simulink model "VRcukie"  (R2013a)
settings: Solver=ode45  StartTime=0.0  StopTime=10.0  RelTol=1e-3
libraries: aerolibanimutils x1, vrlib x1
settings Model: Creator=Grompone  LastModifiedBy=Grompone

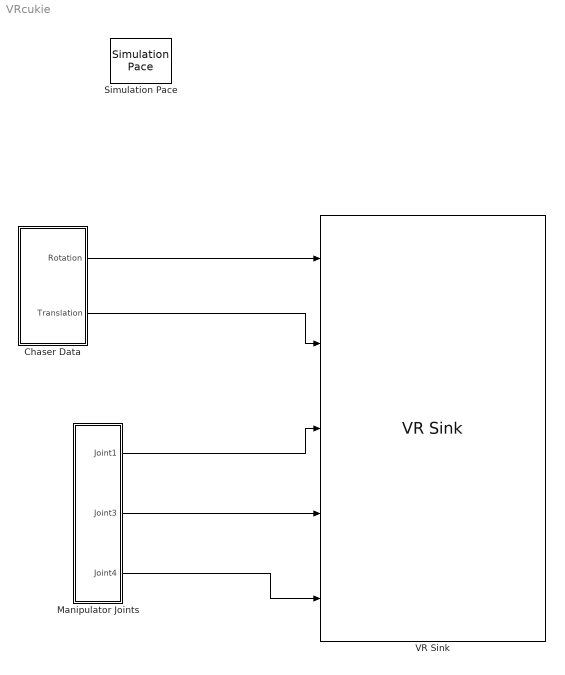
== system VRcukie ==
  Chaser Data : Subsystem
  Manipulator Joints : Subsystem
  Simulation Pace : aerolibanimutils/Simulation Pace  SimulationPace=1  SleepMode=MATLAB Thread  OutputPaceError=off  SampleTime=1/30
      settings: AttributesFormatString=%<SimulationPace> sec/sec
  VR Sink : vrlib/VR Sink  InstantiateOnLoad=on  SampleTime=0.1  ViewEnable=on  RemoteChange=off  RemoteView=off  FieldsWritten=BASE.rotation.4.1.1.double#BASE.translation.3.1.1.double#Joint1.rotation.4.1.1.double#Joint2.rotation.4.1.1.double#Joint3.rotation.4.1.1.double  WorldFileName=C:\Users\Grompone\Dropbox\worknetwork\cukie\Cusakis140505\cukie.wrl  AutoView=off  VideoDimensions=[]  AllowVariableSize=off
  wires:
  Chaser Data/1(Rotation) -> VR Sink/1
  Chaser Data/2(Translation) -> VR Sink/2
  Manipulator Joints/1(Joint1) -> VR Sink/3
  Manipulator Joints/2(Joint3) -> VR Sink/4
  Manipulator Joints/3(Joint4) -> VR Sink/5

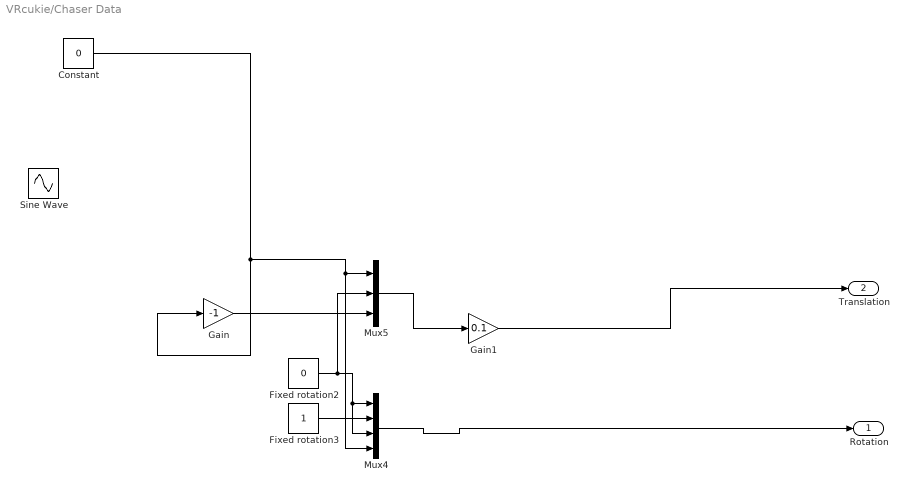
== system VRcukie/Chaser Data ==
  Constant : Constant  Value=0
  Fixed rotation2 : Constant  Value=0
  Fixed rotation3 : Constant
  Gain : Gain  Gain=-1
  Gain1 : Gain  Gain=0.1
  Mux4 : Mux
  Mux5 : Mux  Inputs=3
  Sine Wave : Sin  Amplitude=90  SampleTime=0
  Rotation : Outport
  Translation : Outport  Port=2
  wires:
  Mux5/1 -> Gain1/1
  Fixed rotation2/1 -> Mux4/1, Mux4/3, Mux5/2
  Fixed rotation3/1 -> Mux4/2
  Gain1/1 -> Translation/1
  Mux4/1 -> Rotation/1
  Gain/1 -> Mux5/3
  Constant/1 -> Gain/1, Mux5/1, Mux4/4

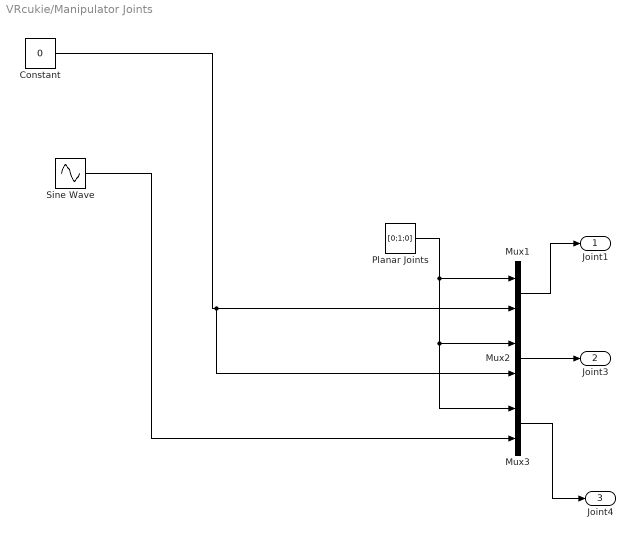
== system VRcukie/Manipulator Joints ==
  Constant : Constant  Value=0
  Mux1 : Mux  Inputs=2
  Mux2 : Mux  Inputs=2
  Mux3 : Mux  Inputs=2
  Planar Joints : Constant  Value=[0;1;0]
  Sine Wave : Sin  SampleTime=0
  Joint1 : Outport
  Joint3 : Outport  Port=2
  Joint4 : Outport  Port=3
  wires:
  Constant/1 -> Mux2/2, Mux1/2
  Planar Joints/1 -> Mux3/1, Mux2/1, Mux1/1
  Mux1/1 -> Joint1/1
  Mux2/1 -> Joint3/1
  Mux3/1 -> Joint4/1
  Sine Wave/1 -> Mux3/2
